simulink model "sysid_system_generate"  (R2015a)
settings: Solver=ode45  StartTime=0.0  StopTime=10  RelTol=1e-3
values from neighbouring files (symbols this model uses):
  Gs = tf([3],[1 3 4])    [sysid_system_generate_m.m]
  h = 0.1    [sysid_system_generate_m.m]
libraries: simulink x1
settings Model: Creator=Steven  LastModifiedBy=Xiaotian

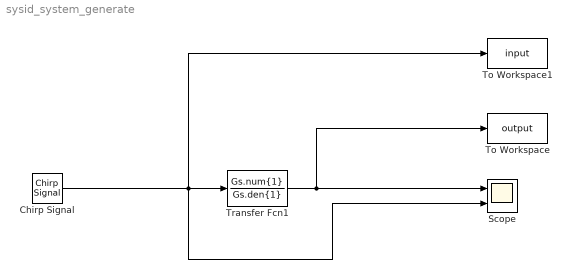
== system sysid_system_generate ==
  Chirp Signal : simulink/Sources/Chirp Signal  f1=0.1  T=10  f2=1
  Scope : Scope  NumInputPorts=2
      settings: TimeRange=20  YMin=-8~-15  YMax=10~15
  To Workspace : ToWorkspace  VariableName=output  SaveFormat=Timeseries  SampleTime=h
  To Workspace1 : ToWorkspace  VariableName=input  SaveFormat=Timeseries  SampleTime=h
  Transfer Fcn1 : TransferFcn  Numerator=Gs.num{1}  Denominator=Gs.den{1}
  wires:
  Chirp Signal/1 -> To Workspace1/1, Scope/2, Transfer Fcn1/1
  Transfer Fcn1/1 -> To Workspace/1, Scope/1
